simulink model "sampleModel1813"  (R2023a)
settings: Solver=VariableStepAuto  StartTime=0.0  StopTime=10.0  RelTol=1e-3
libraries: simulink x3, hdlsllib x2
settings Model: Creator=user1  LastModifiedBy=user1

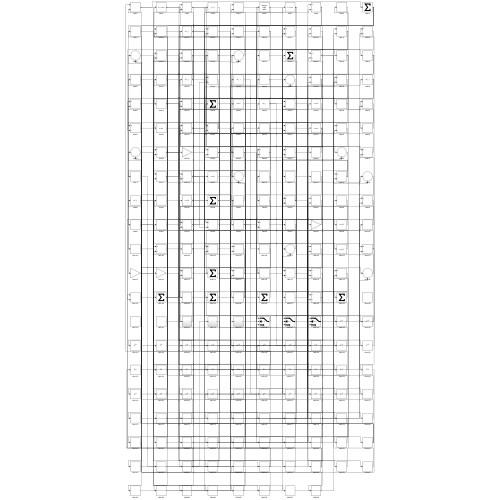
[thumbnail: Simulink's stored preview of the top-level diagram]
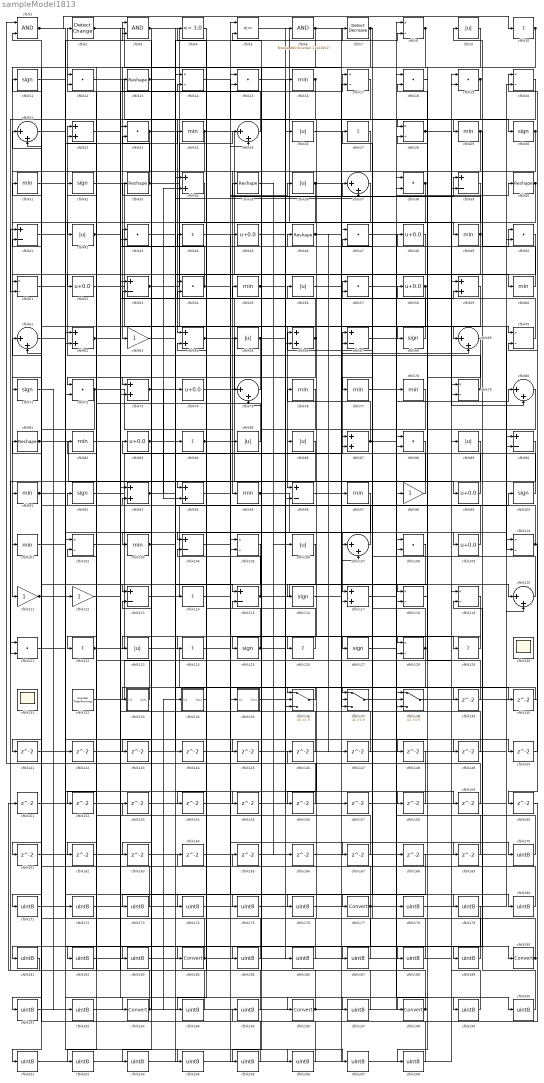
== system sampleModel1813 ==
  cfblk1 : Logic  AllPortsSameDT=off  OutDataTypeStr=boolean
  cfblk{10,27,44,84,114,122,124,126,129} (9 alike) : Sum  Inputs=+
  cfblk{11,30,32,68,71,92,100,116,125,127} (10 alike) : Signum
  cfblk{16,24,29,31,49,55,60,76..78,82,91,95,97,101,103} (16 alike) : MinMax
  cfblk{8,14,17,20,28,51,70,79,102,105,110,118..119,128} (14 alike) : Product  Inputs=*/  RndMeth=Zero  SaturateOnIntegerOverflow=on
  cfblk{39,41,53,67,90,96,104,113,115} (9 alike) : Sum  Inputs=+-
  cfblk{9,26,36,42,56,65,85..86,89,106,123} (11 alike) : Abs  SaturateOnIntegerOverflow=off
  cfblk{21,25,37,61,69,75,80,107,120} (9 alike) : Sum  Inputs=|++
  cfblk{12,15,18..19,23,38,43,47,50,54,57,72,88,108,121} (15 alike) : DotProduct  OutDataTypeStr=Inherit: Inherit via internal rule
  cfblk{45,48,52,58,74,83,99,109} (8 alike) : Bias  Bias=0.0  SaturateOnIntegerOverflow=off
  cfblk{63,98,111..112} (4 alike) : Gain
  cfblk{22,34,59,62,64,66,73,87,93..94,117} (11 alike) : Sum
  cfblk{13,33,35,40,46,81} (6 alike) : Reshape
  cfblk130 : Scope
      settings: Floating=on
  cfblk131 : Scope
      settings: Floating=on
  cfblk132 : hdlsllib/Sources/Counter Free-Running  NumBits=16  tsamp=-1
  cfblk133 : Subsystem
      settings: LibrarySourceBlock=|
      | hdlsllib/Ports &
      | Subsystems/Subsystem
  cfblk134 : Subsystem
      settings: LibrarySourceBlock=|
      | hdlsllib/Ports &
      | Subsystems/Subsystem
  cfblk135 : Subsystem
      settings: LibrarySourceBlock=|
      | hdlsllib/Ports &
      | Subsystems/Subsystem
  cfblk136 : Switch  SaturateOnIntegerOverflow=off  InputSameDT=off
  cfblk137 : Switch  SaturateOnIntegerOverflow=off  InputSameDT=off
  cfblk138 : Switch  SaturateOnIntegerOverflow=off  InputSameDT=off
  cfblk{139..169} (31 alike) : Delay  SampleTime=1
  cfblk{170..176,178..183,185..189,191..192,194..195,197,199..208} (33 alike) : DataTypeConversion  OutDataTypeStr=uint8  SaturateOnIntegerOverflow=off  RndMeth=Floor
  cfblk{177,184,190,193,196,198} (6 alike) : DataTypeConversion  SaturateOnIntegerOverflow=off  RndMeth=Floor
  cfblk2 : simulink/Logic and Bit Operations/Detect Change  vinit=0  OutDataTypeStr=boolean
      settings: LibrarySourceBlock=|
      | hdlsllib/Logic and Bit
      | Operations/Detect
      | Change
  cfblk3 : Logic  AllPortsSameDT=off  OutDataTypeStr=boolean
  cfblk4 : hdlsllib/Logic and Bit Operations/Compare To Constant  relop=<=  const=3.0  OutDataTypeStr=boolean
  cfblk5 : RelationalOperator  Operator=<=  OutDataTypeStr=boolean  InputSameDT=off
  cfblk6 : simulink/Logic and Bit Operations/Bitwise Operator  logicop=AND  UseBitMask=on  BitMask=bin2dec('11011001')  BitMaskRealWorld=Stored Integer
      settings: LibrarySourceBlock=|
      | hdlsllib/Logic and Bit
      | Operations/Bitwise
      | Operator
  cfblk7 : simulink/Logic and Bit Operations/Detect Decrease  vinit=0.0  OutDataTypeStr=boolean
      settings: LibrarySourceBlock=|
      | hdlsllib/Logic and Bit
      | Operations/Detect
      | Decrease
  wires:
  cfblk35/1 -> cfblk106/1
  cfblk115/1 -> cfblk120/1, cfblk54/2
  cfblk34/1 -> cfblk64/1
  cfblk65/1 -> cfblk73/1, cfblk138/3
  cfblk55/1 -> cfblk125/1, cfblk8/2
  cfblk9/1 -> cfblk63/1
  cfblk62/1 -> cfblk46/1, cfblk149/1, cfblk150/1
  cfblk99/1 -> cfblk67/1
  cfblk63/1 -> cfblk58/1
  cfblk30/1 -> cfblk95/1, cfblk71/1
  cfblk71/1 -> cfblk112/1
  cfblk4/1 -> cfblk94/1
  cfblk86/1 -> cfblk122/1
  cfblk37/1 -> cfblk111/1
  cfblk3/1 -> cfblk69/1, cfblk96/2, cfblk163/1
  cfblk87/1 -> cfblk37/1, cfblk76/1, cfblk180/1
  cfblk42/1 -> cfblk158/1, cfblk159/1
  cfblk133/1(Out1) -> cfblk92/1
  cfblk75/1 -> cfblk72/1
  cfblk95/1 -> cfblk117/1, cfblk166/1
  cfblk32/1 -> cfblk96/1
  cfblk76/1 -> cfblk86/1
  cfblk38/1 -> cfblk124/1, cfblk175/1
  cfblk28/1 -> cfblk79/1, cfblk80/2
  cfblk27/1 -> cfblk101/1
  cfblk102/1 -> cfblk184/1
  cfblk58/1 -> cfblk77/1, cfblk118/1
  cfblk33/1 -> cfblk49/1, cfblk23/2
  cfblk98/1 -> cfblk83/1
  cfblk25/1 -> cfblk2/1
  cfblk123/1 -> cfblk136/1
  cfblk64/1 -> cfblk136/2, cfblk26/1
  cfblk74/1 -> cfblk57/1
  cfblk5/1 -> cfblk97/1
  cfblk126/1 -> cfblk55/1
  cfblk23/1 -> cfblk110/1, cfblk162/1
  cfblk46/1 -> cfblk118/2, cfblk147/1
  cfblk122/1 -> cfblk14/1, cfblk48/1, cfblk56/1
  cfblk50/1 -> cfblk75/1
  cfblk125/1 -> cfblk14/2, cfblk104/2, cfblk167/1
  cfblk92/1 -> cfblk87/1
  cfblk116/1 -> cfblk50/1
  cfblk129/1 -> cfblk123/1
  cfblk56/1 -> cfblk67/2
  cfblk111/1 -> cfblk3/1, cfblk192/1
  cfblk96/1 -> cfblk69/2
  cfblk8/1 -> cfblk91/1, cfblk161/1
  cfblk94/1 -> cfblk128/1
  cfblk138/1 -> cfblk20/1
  cfblk84/1 -> cfblk99/1, cfblk36/1
  cfblk119/1 -> cfblk198/1
  cfblk60/1 -> cfblk9/1
  cfblk135/1(Out1) -> cfblk6/1
  cfblk10/1 -> cfblk28/1, cfblk73/2, cfblk57/2, cfblk65/1
  cfblk52/1 -> cfblk98/1
  cfblk14/1 -> cfblk30/1
  cfblk12/1 -> cfblk29/1
  cfblk36/1 -> cfblk72/2, cfblk109/1
  cfblk81/1 -> cfblk128/2, cfblk24/1
  cfblk48/1 -> cfblk126/1
  cfblk70/1 -> cfblk53/2
  cfblk93/1 -> cfblk7/1, cfblk34/2
  cfblk15/1 -> cfblk190/1
  cfblk104/1 -> cfblk39/1
  cfblk120/1 -> cfblk66/1
  cfblk41/1 -> cfblk193/1
  cfblk79/1 -> cfblk22/1, cfblk4/1
  cfblk40/1 -> cfblk103/1, cfblk117/2
  cfblk137/1 -> cfblk38/1
  cfblk49/1 -> cfblk35/1, cfblk152/1
  cfblk128/1 -> cfblk27/1, cfblk156/1
  cfblk6/1 -> cfblk52/1, cfblk139/1
  cfblk68/1 -> cfblk13/1
  cfblk22/1 -> cfblk93/1
  cfblk83/1 -> cfblk59/2, cfblk140/1
  cfblk24/1 -> cfblk78/1, cfblk42/1
  cfblk100/1 -> cfblk18/2
  cfblk132/1 -> cfblk39/2
  cfblk72/1 -> cfblk135/1(In1), cfblk17/1, cfblk171/1
  cfblk85/1 -> cfblk32/1
  cfblk57/1 -> cfblk40/1
  cfblk26/1 -> cfblk129/1
  cfblk13/1 -> cfblk115/1, cfblk60/1
  cfblk45/1 -> cfblk16/1
  cfblk91/1 -> cfblk110/2, cfblk155/1
  cfblk107/1 -> cfblk12/1
  cfblk89/1 -> cfblk177/1
  cfblk1/1 -> cfblk10/1, cfblk206/1
  cfblk113/1 -> cfblk45/1
  cfblk73/1 -> cfblk84/1, cfblk85/1, cfblk94/2
  cfblk82/1 -> cfblk196/1
  cfblk110/1 -> cfblk81/1, cfblk160/1
  cfblk101/1 -> cfblk62/2
  cfblk66/1 -> cfblk43/1, cfblk113/1
  cfblk16/1 -> cfblk43/2, cfblk54/1
  cfblk29/1 -> cfblk185/1, cfblk189/1
  cfblk18/1 -> cfblk68/1
  cfblk20/1 -> cfblk116/1
  cfblk97/1 -> cfblk104/1
  cfblk124/1 -> cfblk5/1
  cfblk88/1 -> cfblk121/2
  cfblk136/1 -> cfblk133/1(In1)
  cfblk109/1 -> cfblk93/2
  cfblk2/1 -> cfblk107/1, cfblk200/1
  cfblk54/1 -> cfblk51/1, cfblk70/1, cfblk3/2
  cfblk53/1 -> cfblk25/1, cfblk37/2
  cfblk19/1 -> cfblk137/3, cfblk51/2
  cfblk7/1 -> cfblk127/1, cfblk173/1
  cfblk127/1 -> cfblk80/1
  cfblk103/1 -> cfblk100/1, cfblk143/1
  cfblk139/1 -> cfblk28/2
  cfblk140/1 -> cfblk137/1
  cfblk59/1 -> cfblk141/1
  cfblk121/1 -> cfblk142/1
  cfblk142/1 -> cfblk137/2
  cfblk143/1 -> cfblk20/2
  cfblk43/1 -> cfblk144/1
  cfblk144/1 -> cfblk18/1
  cfblk51/1 -> cfblk145/1
  cfblk145/1 -> cfblk79/2
  cfblk146/1 -> cfblk64/2
  cfblk147/1 -> cfblk53/1
  cfblk118/1 -> cfblk148/1
  cfblk148/1 -> cfblk1/1
  cfblk149/1 -> cfblk75/2
  cfblk150/1 -> cfblk70/2
  cfblk151/1 -> cfblk38/2
  cfblk152/1 -> cfblk120/2
  cfblk153/1 -> cfblk136/3
  cfblk134/1(Out1) -> cfblk154/1
  cfblk154/1 -> cfblk87/2
  cfblk155/1 -> cfblk66/2
  cfblk156/1 -> cfblk115/2
  cfblk157/1 -> cfblk19/1
  cfblk158/1 -> cfblk1/2
  cfblk159/1 -> cfblk113/2
  cfblk161/1 -> cfblk107/2
  cfblk162/1 -> cfblk22/2
  cfblk163/1 -> cfblk25/2
  cfblk164/1 -> cfblk50/2
  cfblk166/1 -> cfblk17/2
  cfblk167/1 -> cfblk12/2
  cfblk67/1 -> cfblk168/1
  cfblk77/1 -> cfblk169/1
  cfblk169/1 -> cfblk138/1
  cfblk114/1 -> cfblk170/1
  cfblk170/1 -> cfblk88/1
  cfblk171/1 -> cfblk114/1
  cfblk11/1 -> cfblk172/1
  cfblk172/1 -> cfblk88/2
  cfblk173/1 -> cfblk11/1
  cfblk90/1 -> cfblk174/1
  cfblk174/1 -> cfblk138/2
  cfblk175/1 -> cfblk90/1
  cfblk141/1 -> cfblk176/1
  cfblk176/1 -> cfblk90/2
  cfblk177/1 -> cfblk62/1, cfblk183/1
  cfblk47/1 -> cfblk178/1
  cfblk178/1 -> cfblk89/1
  cfblk44/1 -> cfblk179/1
  cfblk180/1 -> cfblk44/1
  cfblk108/1 -> cfblk181/1
  cfblk181/1 -> cfblk151/1
  cfblk39/1 -> cfblk182/1
  cfblk182/1 -> cfblk108/1
  cfblk183/1 -> cfblk108/2
  cfblk184/1 -> cfblk34/1, cfblk59/1
  cfblk185/1 -> cfblk102/1
  cfblk165/1 -> cfblk186/1
  cfblk186/1 -> cfblk102/2
  cfblk21/1 -> cfblk187/1
  cfblk187/1 -> cfblk47/1
  cfblk69/1 -> cfblk188/1
  cfblk188/1 -> cfblk21/1
  cfblk189/1 -> cfblk21/2
  cfblk190/1 -> cfblk146/1, cfblk33/1, cfblk47/2
  cfblk179/1 -> cfblk191/1
  cfblk191/1 -> cfblk15/1
  cfblk192/1 -> cfblk15/2
  cfblk193/1 -> cfblk153/1, cfblk8/1, cfblk134/1(In1), cfblk121/1
  cfblk106/1 -> cfblk194/1
  cfblk194/1 -> cfblk41/1
  cfblk160/1 -> cfblk195/1
  cfblk195/1 -> cfblk41/2
  cfblk196/1 -> cfblk5/2, cfblk23/1
  cfblk112/1 -> cfblk197/1
  cfblk197/1 -> cfblk82/1
  cfblk198/1 -> cfblk165/1, cfblk164/1
  cfblk117/1 -> cfblk199/1
  cfblk199/1 -> cfblk119/1
  cfblk200/1 -> cfblk119/2
  cfblk105/1 -> cfblk201/1
  cfblk201/1 -> cfblk74/1
  cfblk17/1 -> cfblk202/1
  cfblk202/1 -> cfblk105/1
  cfblk168/1 -> cfblk203/1
  cfblk203/1 -> cfblk105/2
  cfblk61/1 -> cfblk204/1
  cfblk204/1 -> cfblk157/1
  cfblk78/1 -> cfblk205/1
  cfblk205/1 -> cfblk61/1
  cfblk206/1 -> cfblk61/2
  cfblk31/1 -> cfblk207/1
  cfblk207/1 -> cfblk19/2
  cfblk80/1 -> cfblk208/1
  cfblk208/1 -> cfblk31/1

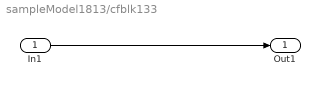
== system sampleModel1813/cfblk133 ==
  In1 : Inport
  Out1 : Outport
  wires:
  In1/1 -> Out1/1

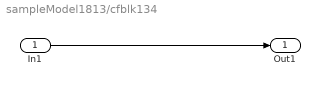
== system sampleModel1813/cfblk134 ==
  In1 : Inport
  Out1 : Outport
  wires:
  In1/1 -> Out1/1

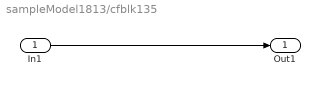
== system sampleModel1813/cfblk135 ==
  In1 : Inport
  Out1 : Outport
  wires:
  In1/1 -> Out1/1
